simulink model "qlabs_qube2_bal_rl"  (R2021a)
settings: Solver=ode1  StartTime=0.0  StopTime=inf  FixedStep=Ts  RelTol=1e-3  EnableMultiTasking=on
undefined symbols (not defined in the file or in its folder): alpha_bal_threshold, B, HIL, q11, q22, q33, q44, qc_get_step_size, r, theta_max, Ts, Vmax
libraries: simulink x4, quarc_library x3, simulink_extras x2, rllib x1
settings Model: ExtModeTrigDuration=5000  Creator=MLevis  LastModifiedBy=MLevis
settings SolverCC: AlgebraicLoopSolver=TrustRegion
settings DataIOCC: ReturnWorkspaceOutputs=off
settings DebuggingCC: UnderspecifiedInitializationDetection=Classic  MergeDetectMultiDrivingBlocksExec=none  SFMachineParentedDataDiag=warning
settings ModelReferenceCC: PropagateSignalLabelsOutOfModel=off
settings SFSimCC: CustomCodeUndefinedFunction=UseInterfaceOnly

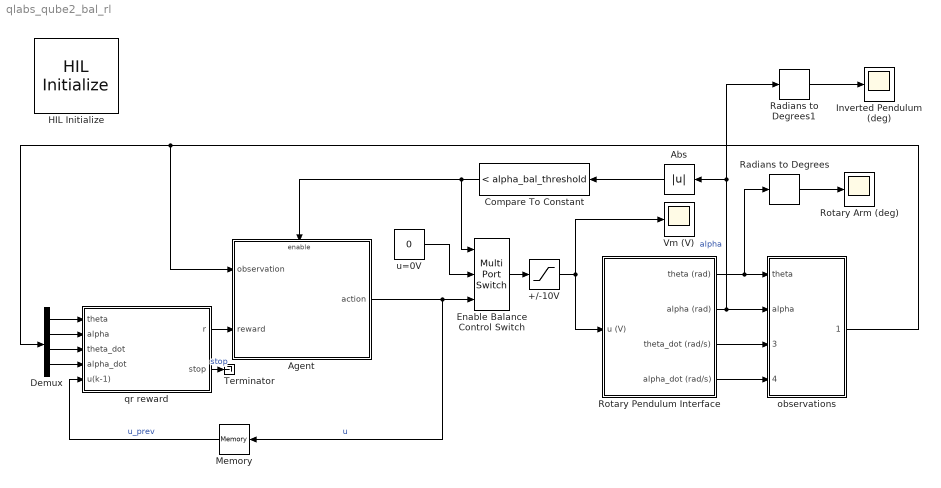
== system qlabs_qube2_bal_rl ==
  +/-10V : Saturate  UpperLimit=10  LowerLimit=-10
  Abs : Abs
  Agent : Subsystem
  Compare To Constant : simulink/Logic and Bit Operations/Compare To Constant  relop=<  const=alpha_bal_threshold  OutDataTypeStr=boolean
  Demux : Demux
  Enable Balance Control Switch : MultiPortSwitch  DataPortOrder=Zero-based contiguous  Inputs=2  zeroidx=on
  HIL Initialize : quarc_library/Data Acquisition/Generic/Configuration/HIL Initialize  object_name=HIL-1  board_type=qube_servo2_usb  board_number=0@tcpip://localhost:18921  board_options=d0=digital;d1=digital;led=auto;update_rate=normal;decimation=1  exclusive=off  active=on  hardware_clocks=[0]  clock_modes=[]  initial_clock_frequencies=[]  set_clock_params_at_start=off  set_clock_params_at_switch_in=off  set_clock_frequencies_at_start=off  set_clock_frequencies_at_switch_in=off  analog_input_channels=[0]  analog_input_configurations=[]  analog_input_maximums=3  analog_input_minimums=-3  set_analog_input_params_at_start=off  set_analog_input_params_at_switch_in=off  analog_output_channels=[0]  analog_output_maximums=15  analog_output_minimums=-15  initial_analog_outputs=[0]  final_analog_outputs=[0]  watchdog_analog_outputs=0  set_analog_output_params_at_start=off  set_analog_output_params_at_switch_in=off  set_analog_outputs_at_start=on  set_analog_outputs_at_switch_in=off  set_analog_outputs_at_terminate=on  set_analog_outputs_at_switch_out=off  set_analog_outputs_on_watchdog=on  digital_input_channels=[]  digital_output_channels=[0]  digital_output_configuration=[]  initial_digital_outputs=[1]  final_digital_outputs=[0]  watchdog_digital_outputs=[0]  set_digital_output_params_at_start=off  set_digital_output_params_at_switch_in=off  set_digital_outputs_at_start=on  set_digital_outputs_at_switch_in=off  set_digital_outputs_at_terminate=on  set_digital_outputs_at_switch_out=off  set_digital_outputs_on_watchdog=on  encoder_channels=[0:1]  quadrature=[4]  encoder_filter_frequency=[]  initial_encoder_counts=[0]  set_encoder_params_at_start=off  set_encoder_params_at_switch_in=off  set_encoder_counts_at_start=on  set_encoder_counts_at_switch_in=off  pwm_channels=[]  pwm_modes=[]  pwm_frequency=[]  pwm_configuration=[]  pwm_alignment=[]  pwm_polarity=[]  pwm_leading_deadband=[]  pwm_trailing_deadband=[]  initial_pwm_outputs=[]  final_pwm_outputs=[]  watchdog_pwm_outputs=[]  set_pwm_params_at_start=off  set_pwm_params_at_switch_in=off  set_pwm_outputs_at_start=off  set_pwm_outputs_at_switch_in=off  set_pwm_outputs_at_terminate=off  set_pwm_outputs_at_switch_out=off  set_pwm_outputs_on_watchdog=off  other_output_channels=[11000:11002]  initial_other_outputs=[0 1 0]  final_other_outputs=[1 0 0]  watchdog_other_outputs=[0 0 1]  set_other_outputs_at_start=on  set_other_outputs_at_switch_in=off  set_other_outputs_at_terminate=on  set_other_outputs_at_switch_out=off  set_other_outputs_on_watchdog=on
  Inverted Pendulum (deg) : Scope
  Memory : Memory
  Radians to Degrees : simulink_extras/Transformations/Radians to Degrees
  Radians to Degrees1 : simulink_extras/Transformations/Radians to Degrees
  Rotary Arm (deg) : Scope
  Rotary Pendulum Interface : Subsystem
  Terminator : Terminator
  Vm (V) : Scope
  observations : Subsystem  VariantControl=sincos
  qr reward : Subsystem
  u=0V : Constant  Value=0
  wires:
  Radians to Degrees/1 -> Rotary Arm (deg)/1
  Radians to Degrees1/1 -> Inverted Pendulum (deg)/1
  +/-10V/1 -> Rotary Pendulum Interface/1(u (V)), Vm (V)/1
  Rotary Pendulum Interface/1(theta (rad)) -> observations/1(theta), Radians to Degrees/1
  Rotary Pendulum Interface/3(theta_dot (rad/s)) -> observations/3(theta_dot)
  Rotary Pendulum Interface/4(alpha_dot (rad/s)) -> observations/4(alpha_dot)
  Memory/1 -> qr reward/5(u(k-1))  "u_prev"
  observations/1(observations) -> Agent/1(observation), Demux/1
  qr reward/1(r) -> Agent/2(reward)
  Demux/1 -> qr reward/1(theta)
  Demux/2 -> qr reward/2(alpha)
  Demux/3 -> qr reward/3(theta_dot)
  Demux/4 -> qr reward/4(alpha_dot)
  qr reward/2(stop) -> Terminator/1  "stop"
  Compare To Constant/1 -> Enable Balance Control Switch/1, Agent/Enable
  Rotary Pendulum Interface/2(alpha (rad)) -> Radians to Degrees1/1, Abs/1, observations/2(alpha)  "alpha"
  Abs/1 -> Compare To Constant/1
  Enable Balance Control Switch/1 -> +/-10V/1
  Agent/1(action) -> Memory/1, Enable Balance Control Switch/3  "u"
  u=0V/1 -> Enable Balance Control Switch/2

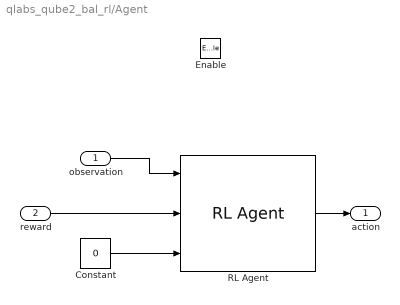
== system qlabs_qube2_bal_rl/Agent ==
  observation : Inport
  reward : Inport  Port=2
  Enable : EnablePort
  Constant : Constant  Value=0  SampleTime=Ts
  RL Agent : rllib/RL Agent  Agent=agent  ExternalActionAsInput=off  ProvideCumRwd=off  TreatAsDirectFeedthrough=on
  action : Outport  InitialOutput=[0]
  wires:
  observation/1 -> RL Agent/1
  RL Agent/1 -> action/1
  reward/1 -> RL Agent/2
  Constant/1 -> RL Agent/3

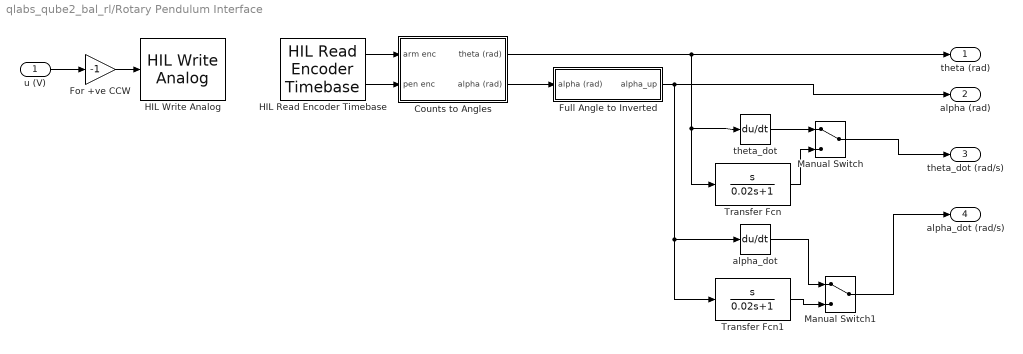
== system qlabs_qube2_bal_rl/Rotary Pendulum Interface ==
  u (V) : Inport
  Counts to Angles : Subsystem
  For +ve CCW : Gain  Gain=-1
  Full Angle to Inverted : Subsystem
  HIL Read Encoder Timebase : quarc_library/Data Acquisition/Generic/Timebases/HIL Read Encoder Timebase  object_name=HIL-1  clock=0  channels=[0:1]  active=on  vector_output=off  data_type_mode=Inherit via back propagation  data_type=double  overflow_mode=Synchronize (for simulated cards only)  samples_in_buffer=max(ceil(1/qc_get_step_size), 1)
  HIL Write Analog : quarc_library/Data Acquisition/Generic/Immediate I//O/HIL Write Analog  object_name=HIL-1  channels=0  sample_time=-1  active=on  vector_input=off
  Manual Switch : ManualSwitch
  Manual Switch1 : ManualSwitch
  Transfer Fcn : TransferFcn  Numerator=[1 0]  Denominator=[0.02 1]
  Transfer Fcn1 : TransferFcn  Numerator=[1 0]  Denominator=[0.02 1]
  alpha_dot : Derivative
  theta_dot : Derivative
  theta (rad) : Outport  VectorParamsAs1DForOutWhenUnconnected=off
  alpha (rad) : Outport  Port=2  VectorParamsAs1DForOutWhenUnconnected=off
  theta_dot (rad/s) : Outport  Port=3  VectorParamsAs1DForOutWhenUnconnected=off
  alpha_dot (rad/s) : Outport  Port=4  VectorParamsAs1DForOutWhenUnconnected=off
  wires:
  For +ve CCW/1 -> HIL Write Analog/1
  u (V)/1 -> For +ve CCW/1
  HIL Read Encoder Timebase/1 -> Counts to Angles/1(arm enc)
  HIL Read Encoder Timebase/2 -> Counts to Angles/2(pen enc)
  Counts to Angles/1(theta (rad)) -> theta (rad)/1, theta_dot/1, Transfer Fcn/1
  Counts to Angles/2(alpha (rad)) -> Full Angle to Inverted/1(alpha (rad))
  Full Angle to Inverted/1(alpha_up) -> alpha (rad)/1, alpha_dot/1, Transfer Fcn1/1
  theta_dot/1 -> Manual Switch/1
  Transfer Fcn/1 -> Manual Switch/2
  alpha_dot/1 -> Manual Switch1/1
  Transfer Fcn1/1 -> Manual Switch1/2
  Manual Switch1/1 -> alpha_dot (rad/s)/1
  Manual Switch/1 -> theta_dot (rad/s)/1

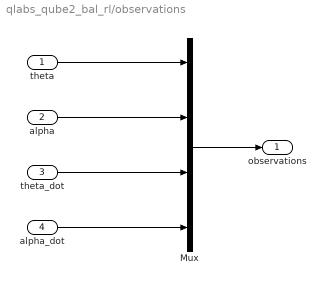
== system qlabs_qube2_bal_rl/observations ==
  theta : Inport
  alpha : Inport  Port=2
  theta_dot : Inport  Port=3
  alpha_dot : Inport  Port=4
  Mux : Mux
  observations : Outport  VectorParamsAs1DForOutWhenUnconnected=off
  wires:
  alpha_dot/1 -> Mux/4
  theta_dot/1 -> Mux/3
  alpha/1 -> Mux/2
  theta/1 -> Mux/1
  Mux/1 -> observations/1

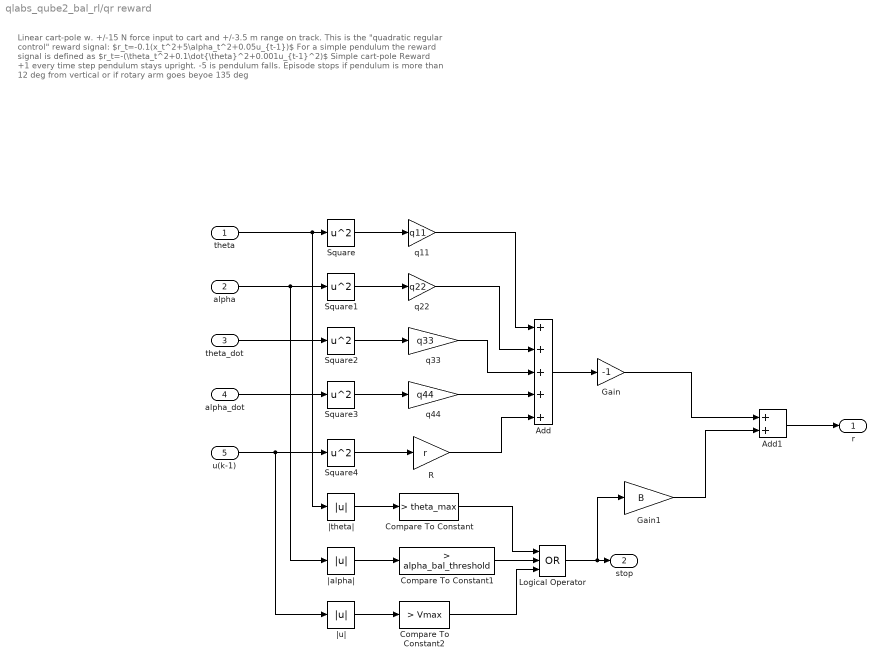
== system qlabs_qube2_bal_rl/qr reward ==
  note: Linear cart-pole w. +/-15 N force input to cart and +/-3.5 m range on track. This is the "quadratic regular control" reward signal:
      | $r_t=-0.1(x_t^2+5\alpha_t^2+0.05u_{t-1})$
      | For a simple pendulum the reward signal is defined as
      | $r_t=-(\theta_t^2+0.1\dot{\theta}^2+0.001u_{t-1}^2)$
      | Simple cart-pole
      | Reward +1 every time step pendulum stays upright. -5 is pendulum falls.
      | Episode stops if pendulum is more than 12 deg from vertical or if rotary arm goes beyoe 135 deg
  theta : Inport
  alpha : Inport  Port=2
  theta_dot : Inport  Port=3
  alpha_dot : Inport  Port=4
  u(k-1) : Inport  Port=5
  Add : Sum  Inputs=+++++
  Add1 : Sum
  Compare To Constant : simulink/Logic and Bit Operations/Compare To Constant  relop=>  const=theta_max  OutDataTypeStr=boolean
  Compare To Constant1 : simulink/Logic and Bit Operations/Compare To Constant  relop=>  const=alpha_bal_threshold  OutDataTypeStr=boolean
  Compare To Constant2 : simulink/Logic and Bit Operations/Compare To Constant  relop=>  const=Vmax  OutDataTypeStr=boolean
  Gain : Gain  Gain=-1
  Gain1 : Gain  Gain=B
  Logical Operator : Logic  Operator=OR  Inputs=3  AllPortsSameDT=off  OutDataTypeStr=boolean
  R : Gain  Gain=r
  Square{,1..4} (5 alike) : Math  Operator=square  SaturateOnIntegerOverflow=on
  q11 : Gain  Gain=q11
  q22 : Gain  Gain=q22
  q33 : Gain  Gain=q33
  q44 : Gain  Gain=q44
  |alpha| : Abs
  |theta| : Abs
  |u| : Abs
  r : Outport  VectorParamsAs1DForOutWhenUnconnected=off
  stop : Outport  Port=2  VectorParamsAs1DForOutWhenUnconnected=off
  wires:
  Add1/1 -> r/1
  Gain1/1 -> Add1/2
  Gain/1 -> Add1/1
  Compare To Constant1/1 -> Logical Operator/2
  Compare To Constant2/1 -> Logical Operator/3
  Add/1 -> Gain/1
  q44/1 -> Add/4
  q22/1 -> Add/2
  q33/1 -> Add/3
  q11/1 -> Add/1
  R/1 -> Add/5
  |u|/1 -> Compare To Constant2/1
  Square4/1 -> R/1
  u(k-1)/1 -> |u|/1, Square4/1
  Square3/1 -> q44/1
  alpha_dot/1 -> Square3/1
  theta_dot/1 -> Square2/1
  Square2/1 -> q33/1
  Square1/1 -> q22/1
  Square/1 -> q11/1
  Logical Operator/1 -> stop/1, Gain1/1
  |alpha|/1 -> Compare To Constant1/1
  alpha/1 -> |alpha|/1, Square1/1
  Compare To Constant/1 -> Logical Operator/1
  theta/1 -> |theta|/1, Square/1
  |theta|/1 -> Compare To Constant/1

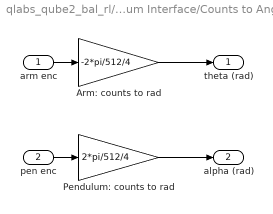
== system qlabs_qube2_bal_rl/Rotary Pendulum Interface/Counts to Angles ==
  arm enc : Inport
  pen enc : Inport  Port=2
  Arm: counts to rad : Gain  Gain=-2*pi/512/4
  Pendulum: counts to rad : Gain  Gain=2*pi/512/4
  theta (rad) : Outport  VectorParamsAs1DForOutWhenUnconnected=off
  alpha (rad) : Outport  Port=2  VectorParamsAs1DForOutWhenUnconnected=off
  wires:
  pen enc/1 -> Pendulum: counts to rad/1
  arm enc/1 -> Arm: counts to rad/1
  Arm: counts to rad/1 -> theta (rad)/1
  Pendulum: counts to rad/1 -> alpha (rad)/1

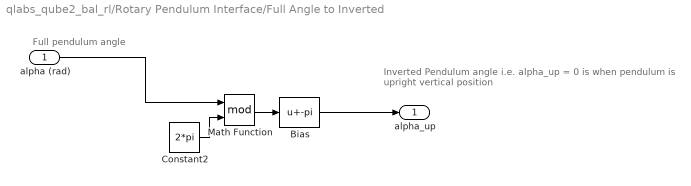
== system qlabs_qube2_bal_rl/Rotary Pendulum Interface/Full Angle to Inverted ==
  note: Full pendulum angle
  note: Inverted Pendulum angle
      | i.e. alpha_up = 0 is when pendulum is upright vertical position
  alpha (rad) : Inport
  Bias : Bias  Bias=-pi
  Constant2 : Constant  Value=2*pi
  Math Function : Math  Operator=mod  SignedPower=on  SaturateOnIntegerOverflow=on
  alpha_up : Outport  VectorParamsAs1DForOutWhenUnconnected=off
  wires:
  Math Function/1 -> Bias/1
  alpha (rad)/1 -> Math Function/1
  Bias/1 -> alpha_up/1
  Constant2/1 -> Math Function/2
